simulink model "BLDCmotorControl_FOC_R2017b"  (R2017b)
settings: Solver=FixedStepDiscrete  StartTime=0  StopTime=1  FixedStep=Ts  MaxStep=1e-6  RelTol=1e-6  AbsTol=1e-6  EnableMultiTasking=on
PreLoadFcn:
  | addpath(genpath('01_Libraries'));
  | addpath(genpath('02_Figures'));
InitFcn:
  | init_model;
values from neighbouring files (symbols this model uses):
  a_elecAngle = 60    [init_model_Ffwd.m]
  a_elecPeriod = 360    [init_model_Ffwd.m]
  b_DCLinkCurrAvail = 0    [init_model_Ffwd.m]
  b_selPhaABCurrMeas = 1    [init_model_Ffwd.m]
  cf_speedCoef = round(f_ctrl * a_mechAngle * (pi/180) * (30/pi))    [init_model_Ffwd.m]
  i_thresOutlier = 200    [init_model_Ffwd.m]
  n_commAcvLo = 15    [init_model_Ffwd.m]
  n_commDeacvHi = 30    [init_model_Ffwd.m]
  r_sin_M1 = sin((a_elecAngle_XA + 30)*(pi/180))    [init_model_Ffwd.m]
  r_whl = 6.5 * 2.54 * 1e-2 / 2    (= 0.08255)    [init_model_Ffwd.m]
  res_elecAngle = 2    [init_model_Ffwd.m]
  Ts = 5e-6    (= 5e-06)    [init_model_Ffwd.m]    (also in pe_electric_engine_dyno_data.m = 1e-05)
  Ts_ctrl = 6e-5    (= 6e-05)    [init_model_Ffwd.m]
  vec_hallToPos = [0 2 0 1 4 3 5 0]    [init_model_Ffwd.m]
  z_commutMap_M1 = [-1 -1  0  1  1  0 ... (first row only)    [init_model_Ffwd.m]
  z_ctrlTypSel = 1    [init_model_Ffwd.m]
  z_maxCntRst = 2000    [init_model_Ffwd.m]
undefined symbols (not defined in the file or in its folder): a_phaAdv_M1, b_phaAdvEna, CTRL_COMM, DiscIntNeverNeededParam, Down, dz_counterHi, dz_counterLo, Kb_Id, Kb_Iq, Kb_n, Ki_Id, Ki_Iq, Ki_n, Kp_Id, Kp_Iq, Kp_n, n_motPhaAdvEna, r_commDCDeacv, sigbuilder_block, Up, V_circleLim_M1, V_max, V_min
libraries: pePwmGenerator x7, BLDC_controller_Lib x6, powerlib x6, simulink x5
(part 3 of 3)

== system BLDCmotorControl_FOC_R2017b/BLDC_controller/BLDC_controller/F03_Field_Oriented_Control/Clarke_Transform/Clarke_PhasesAB ==
  note: Clarke Transform:
      | i_alpha = i_phaA
      | i_beta = ((1/sqrt(3))*i_phaA + (2/sqrt(3))*i_phaB)
  i_phaA : Inport
  i_phaB : Inport  Port=2
  Action Port : ActionPort  ActionType=then
  Gain1 : Gain  Tag=struct('comment',struct('text','','placement',1),'logdata',struct('maxnumvals',inf,'plotchannels',[],'loggingmode',3,'channels',1),'output',struct('variable','','description','','name','$S_$B','width',1,'address','','max',NaN,'min',NaN,'class','default','type','CONTINUOUS','scaling','','lsb',1,'offset',0,'arb',0,'freeze',1,'unit','','autoscalingmode',1,'lowerheadroom',1,'upperheadroom',1,'headroomunit','bit','keepdatatype',1,'checkmin',0,'checkmax',0,'castoutput',0,'show',0),'gain',struct('variable','','description','','name','$S_$B_gain','width',1,'address','','max',NaN,'min',NaN,'class','default','type','CONTINUOUS','scaling','','lsb',1,'offset',0,'arb',0,'freeze',1,'unit','','keepdatatype',1,'value','1','scalar',0,'tolerance',1),'scalingvalid',0,'date',730486)  Gain=2/sqrt(3)  RndMeth=Zero
  Gain3 : Gain  Tag=struct('comment',struct('text','','placement',1),'logdata',struct('maxnumvals',inf,'plotchannels',[],'loggingmode',3,'channels',1),'output',struct('variable','','description','','name','$S_$B','width',1,'address','','max',NaN,'min',NaN,'class','default','type','CONTINUOUS','scaling','','lsb',1,'offset',0,'arb',0,'freeze',1,'unit','','autoscalingmode',1,'lowerheadroom',1,'upperheadroom',1,'headroomunit','bit','keepdatatype',1,'checkmin',0,'checkmax',0,'castoutput',0,'show',0),'gain',struct('variable','','description','','name','$S_$B_gain','width',1,'address','','max',NaN,'min',NaN,'class','default','type','CONTINUOUS','scaling','','lsb',1,'offset',0,'arb',0,'freeze',1,'unit','','keepdatatype',1,'value','1','scalar',0,'tolerance',1),'scalingvalid',0,'date',730486)  Gain=1/sqrt(3)  RndMeth=Zero
  Sum6 : Sum  RndMeth=Simplest
  for_merge : Gain  Tag=struct('comment',struct('text','','placement',1),'logdata',struct('maxnumvals',inf,'plotchannels',[],'loggingmode',3,'channels',1),'output',struct('variable','','description','','name','$S_$B','width',1,'address','','max',NaN,'min',NaN,'class','default','type','CONTINUOUS','scaling','','lsb',1,'offset',0,'arb',0,'freeze',1,'unit','','autoscalingmode',1,'lowerheadroom',1,'upperheadroom',1,'headroomunit','bit','keepdatatype',1,'checkmin',0,'checkmax',0,'castoutput',0,'show',0),'gain',struct('variable','','description','','name','$S_$B_gain','width',1,'address','','max',NaN,'min',NaN,'class','default','type','CONTINUOUS','scaling','','lsb',1,'offset',0,'arb',0,'freeze',1,'unit','','keepdatatype',1,'value','1','scalar',0,'tolerance',1),'scalingvalid',0,'date',730486)  RndMeth=Zero
  i_alphaAB : Outport
  i_betaAB : Outport  Port=2
  wires:
  i_phaB/1 -> [i_phaB]
  i_phaA/1 -> [i_phaA]
  [i_phaB] -> Gain1/1
  [i_phaA] -> for_merge/1, Gain3/1
  Gain3/1 -> Sum6/1
  Sum6/1 -> i_betaAB/1  "beta"
  Gain1/1 -> Sum6/2
  for_merge/1 -> i_alphaAB/1

== system BLDCmotorControl_FOC_R2017b/BLDC_controller/BLDC_controller/F03_Field_Oriented_Control/Clarke_Transform/Clarke_PhasesBC ==
  note: Clarke Transform:
      | i_alpha = - i_phaB - i_phaC
      | i_beta = (1/sqrt(3)) * (i_phaB - i_phaC)
  i_phaB : Inport
  i_phaC : Inport  Port=2
  Action Port : ActionPort  ActionType=else
  Gain2 : Gain  Tag=struct('comment',struct('text','','placement',1),'logdata',struct('maxnumvals',inf,'plotchannels',[],'loggingmode',3,'channels',1),'output',struct('variable','','description','','name','$S_$B','width',1,'address','','max',NaN,'min',NaN,'class','default','type','CONTINUOUS','scaling','','lsb',1,'offset',0,'arb',0,'freeze',1,'unit','','autoscalingmode',1,'lowerheadroom',1,'upperheadroom',1,'headroomunit','bit','keepdatatype',1,'checkmin',0,'checkmax',0,'castoutput',0,'show',0),'gain',struct('variable','','description','','name','$S_$B_gain','width',1,'address','','max',NaN,'min',NaN,'class','default','type','CONTINUOUS','scaling','','lsb',1,'offset',0,'arb',0,'freeze',1,'unit','','keepdatatype',1,'value','1','scalar',0,'tolerance',1),'scalingvalid',0,'date',730486)  Gain=1/sqrt(3)  RndMeth=Zero
  Sum1 : Sum  Inputs=--  RndMeth=Simplest
  Sum2 : Sum  Inputs=+-  RndMeth=Simplest
  i_alphaBC : Outport
  i_betaBC : Outport  Port=2
  wires:
  [i_phaC] -> Sum1/2
  [i_phaB] -> Sum1/1
  [i_phaC] -> Sum2/2
  Gain2/1 -> i_betaBC/1
  Sum2/1 -> Gain2/1
  [i_phaB] -> Sum2/1
  Sum1/1 -> i_alphaBC/1
  i_phaB/1 -> [i_phaB]
  i_phaC/1 -> [i_phaC]

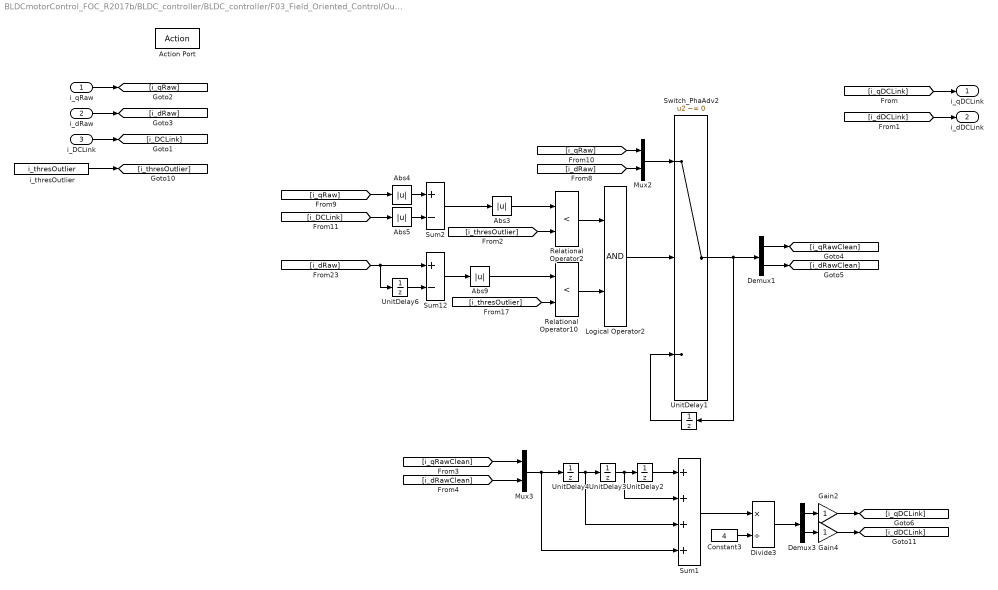
== system BLDCmotorControl_FOC_R2017b/BLDC_controller/BLDC_controller/F03_Field_Oriented_Control/Outliers_Removal/DCLink_Current_Available ==
  i_qRaw : Inport
  i_dRaw : Inport  Port=2
  i_DCLink : Inport  Port=3
  Action Port : ActionPort  ActionType=then
  Abs{3..5,9} (4 alike) : Abs
  Constant3 : Constant  Value=4  OutDataTypeStr=Inherit: Inherit via back propagation
  Demux1 : Demux  Outputs=2
  Demux3 : Demux  Outputs=2
  Divide3 : Product  Inputs=*/  RndMeth=Simplest
  Gain2 : Gain  Tag=struct('comment',struct('text','','placement',1),'logdata',struct('maxnumvals',inf,'plotchannels',[],'loggingmode',3,'channels',1),'output',struct('variable','','description','','name','$S_$B','width',1,'address','','max',NaN,'min',NaN,'class','default','type','CONTINUOUS','scaling','','lsb',1,'offset',0,'arb',0,'freeze',1,'unit','','autoscalingmode',1,'lowerheadroom',1,'upperheadroom',1,'headroomunit','bit','keepdatatype',1,'checkmin',0,'checkmax',0,'castoutput',0,'show',0),'gain',struct('variable','','description','','name','$S_$B_gain','width',1,'address','','max',NaN,'min',NaN,'class','default','type','CONTINUOUS','scaling','','lsb',1,'offset',0,'arb',0,'freeze',1,'unit','','keepdatatype',1,'value','1','scalar',0,'tolerance',1),'scalingvalid',0,'date',730486)  RndMeth=Zero  SaturateOnIntegerOverflow=on  OutDataTypeStr=Inherit: Same as input  ParamDataTypeStr=Inherit: Same as input
  Gain4 : Gain  Tag=struct('comment',struct('text','','placement',1),'logdata',struct('maxnumvals',inf,'plotchannels',[],'loggingmode',3,'channels',1),'output',struct('variable','','description','','name','$S_$B','width',1,'address','','max',NaN,'min',NaN,'class','default','type','CONTINUOUS','scaling','','lsb',1,'offset',0,'arb',0,'freeze',1,'unit','','autoscalingmode',1,'lowerheadroom',1,'upperheadroom',1,'headroomunit','bit','keepdatatype',1,'checkmin',0,'checkmax',0,'castoutput',0,'show',0),'gain',struct('variable','','description','','name','$S_$B_gain','width',1,'address','','max',NaN,'min',NaN,'class','default','type','CONTINUOUS','scaling','','lsb',1,'offset',0,'arb',0,'freeze',1,'unit','','keepdatatype',1,'value','1','scalar',0,'tolerance',1),'scalingvalid',0,'date',730486)  RndMeth=Zero  SaturateOnIntegerOverflow=on  OutDataTypeStr=Inherit: Same as input  ParamDataTypeStr=Inherit: Same as input
  Logical Operator2 : Logic  AllPortsSameDT=off  OutDataTypeStr=boolean
  Mux2 : Mux  Inputs=2
  Mux3 : Mux  Inputs=2
  Relational Operator10 : RelationalOperator  Operator=<  OutDataTypeStr=boolean  RndMeth=Simplest
  Relational Operator2 : RelationalOperator  Operator=<  OutDataTypeStr=boolean  RndMeth=Simplest
  Sum1 : Sum  Inputs=++++  RndMeth=Simplest  InputSameDT=on
  Sum12 : Sum  Inputs=+-  RndMeth=Simplest
  Sum2 : Sum  Inputs=+-  RndMeth=Simplest
  Switch_PhaAdv2 : Switch  Criteria=u2 ~= 0  OutDataTypeStr=Inherit: Inherit via back propagation  RndMeth=Zero
  UnitDelay{1..4,6} (5 alike) : UnitDelay  SampleTime=-1
  i_thresOutlier : Constant  Value=i_thresOutlier  OutDataTypeStr=Inherit: Inherit via back propagation
  i_qDCLink : Outport
  i_dDCLink : Outport  Port=2
  wires:
  [i_dDCLink] -> i_dDCLink/1
  i_qRaw/1 -> [i_qRaw]
  [i_qDCLink] -> i_qDCLink/1
  i_dRaw/1 -> [i_dRaw]
  i_DCLink/1 -> [i_DCLink]
  Switch_PhaAdv2/1 -> Demux1/1, UnitDelay1/1
  Mux2/1 -> Switch_PhaAdv2/1
  Logical Operator2/1 -> Switch_PhaAdv2/2
  [i_DCLink] -> Abs5/1
  UnitDelay6/1 -> Sum12/2
  Demux1/1 -> [i_qRawClean]
  [i_thresOutlier] -> Relational Operator2/2
  Relational Operator10/1 -> Logical Operator2/2
  [i_dRaw] -> Mux2/2
  Abs9/1 -> Relational Operator10/1
  [i_thresOutlier] -> Relational Operator10/2
  Abs5/1 -> Sum2/2
  [i_dRaw] -> UnitDelay6/1, Sum12/1
  Abs3/1 -> Relational Operator2/1
  Demux1/2 -> [i_dRawClean]
  UnitDelay1/1 -> Switch_PhaAdv2/3
  [i_qRaw] -> Abs4/1
  [i_qRaw] -> Mux2/1
  Abs4/1 -> Sum2/1
  Relational Operator2/1 -> Logical Operator2/1
  Sum2/1 -> Abs3/1
  Sum12/1 -> Abs9/1
  Demux3/2 -> Gain4/1
  Gain2/1 -> [i_qDCLink]
  Divide3/1 -> Demux3/1
  Mux3/1 -> Sum1/4, UnitDelay4/1
  Gain4/1 -> [i_dDCLink]
  UnitDelay4/1 -> Sum1/3, UnitDelay3/1
  [i_qRawClean] -> Mux3/1
  Sum1/1 -> Divide3/1
  UnitDelay3/1 -> Sum1/2, UnitDelay2/1
  Constant3/1 -> Divide3/2
  UnitDelay2/1 -> Sum1/1
  Demux3/1 -> Gain2/1
  [i_dRawClean] -> Mux3/2
  i_thresOutlier/1 -> [i_thresOutlier]

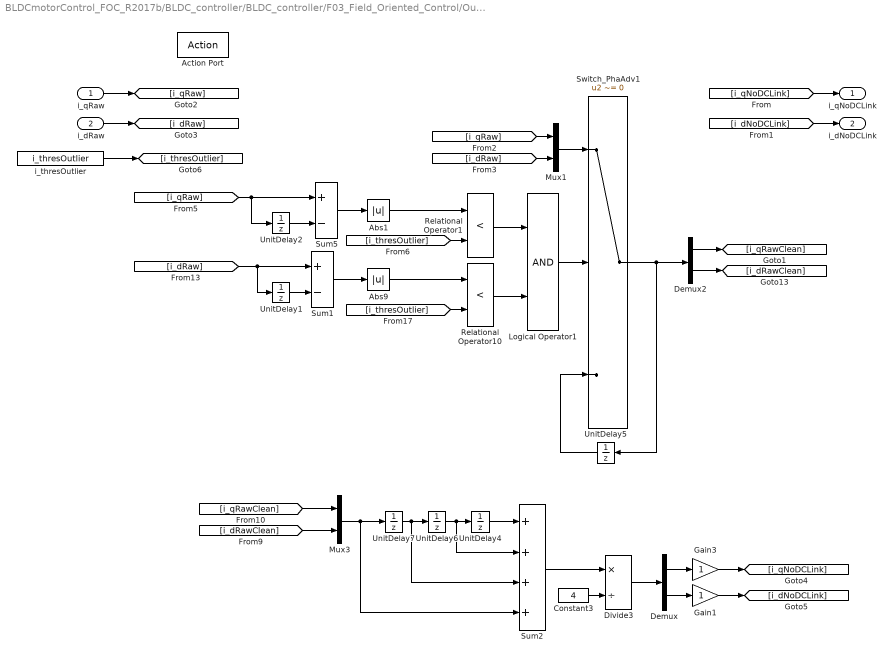
== system BLDCmotorControl_FOC_R2017b/BLDC_controller/BLDC_controller/F03_Field_Oriented_Control/Outliers_Removal/DCLink_Current_Not_Available ==
  i_qRaw : Inport
  i_dRaw : Inport  Port=2
  Action Port : ActionPort  ActionType=else
  Abs1 : Abs
  Abs9 : Abs
  Constant3 : Constant  Value=4  OutDataTypeStr=Inherit: Inherit via back propagation
  Demux : Demux  Outputs=2
  Demux2 : Demux  Outputs=2
  Divide3 : Product  Inputs=*/  RndMeth=Simplest
  Gain1 : Gain  Tag=struct('comment',struct('text','','placement',1),'logdata',struct('maxnumvals',inf,'plotchannels',[],'loggingmode',3,'channels',1),'output',struct('variable','','description','','name','$S_$B','width',1,'address','','max',NaN,'min',NaN,'class','default','type','CONTINUOUS','scaling','','lsb',1,'offset',0,'arb',0,'freeze',1,'unit','','autoscalingmode',1,'lowerheadroom',1,'upperheadroom',1,'headroomunit','bit','keepdatatype',1,'checkmin',0,'checkmax',0,'castoutput',0,'show',0),'gain',struct('variable','','description','','name','$S_$B_gain','width',1,'address','','max',NaN,'min',NaN,'class','default','type','CONTINUOUS','scaling','','lsb',1,'offset',0,'arb',0,'freeze',1,'unit','','keepdatatype',1,'value','1','scalar',0,'tolerance',1),'scalingvalid',0,'date',730486)  RndMeth=Zero  SaturateOnIntegerOverflow=on  OutDataTypeStr=Inherit: Same as input  ParamDataTypeStr=Inherit: Same as input
  Gain3 : Gain  Tag=struct('comment',struct('text','','placement',1),'logdata',struct('maxnumvals',inf,'plotchannels',[],'loggingmode',3,'channels',1),'output',struct('variable','','description','','name','$S_$B','width',1,'address','','max',NaN,'min',NaN,'class','default','type','CONTINUOUS','scaling','','lsb',1,'offset',0,'arb',0,'freeze',1,'unit','','autoscalingmode',1,'lowerheadroom',1,'upperheadroom',1,'headroomunit','bit','keepdatatype',1,'checkmin',0,'checkmax',0,'castoutput',0,'show',0),'gain',struct('variable','','description','','name','$S_$B_gain','width',1,'address','','max',NaN,'min',NaN,'class','default','type','CONTINUOUS','scaling','','lsb',1,'offset',0,'arb',0,'freeze',1,'unit','','keepdatatype',1,'value','1','scalar',0,'tolerance',1),'scalingvalid',0,'date',730486)  RndMeth=Zero  SaturateOnIntegerOverflow=on  OutDataTypeStr=Inherit: Same as input  ParamDataTypeStr=Inherit: Same as input
  Logical Operator1 : Logic  AllPortsSameDT=off  OutDataTypeStr=boolean
  Mux1 : Mux  Inputs=2
  Mux3 : Mux  Inputs=2
  Relational Operator1 : RelationalOperator  Operator=<  OutDataTypeStr=boolean  RndMeth=Simplest
  Relational Operator10 : RelationalOperator  Operator=<  OutDataTypeStr=boolean  RndMeth=Simplest
  Sum1 : Sum  Inputs=+-  RndMeth=Simplest
  Sum2 : Sum  Inputs=++++  RndMeth=Simplest  InputSameDT=on
  Sum5 : Sum  Inputs=+-  RndMeth=Simplest
  Switch_PhaAdv1 : Switch  Criteria=u2 ~= 0  OutDataTypeStr=Inherit: Inherit via back propagation  RndMeth=Zero
  UnitDelay{1..2,4..7} (6 alike) : UnitDelay  SampleTime=-1
  i_thresOutlier : Constant  Value=i_thresOutlier  OutDataTypeStr=Inherit: Inherit via back propagation
  i_qNoDCLink : Outport
  i_dNoDCLink : Outport  Port=2
  wires:
  i_qRaw/1 -> [i_qRaw]
  i_dRaw/1 -> [i_dRaw]
  [i_qNoDCLink] -> i_qNoDCLink/1
  [i_dNoDCLink] -> i_dNoDCLink/1
  Logical Operator1/1 -> Switch_PhaAdv1/2
  Constant3/1 -> Divide3/2
  UnitDelay6/1 -> Sum2/2, UnitDelay4/1
  UnitDelay7/1 -> Sum2/3, UnitDelay6/1
  [i_qRawClean] -> Mux3/1
  Sum1/1 -> Abs9/1
  Abs9/1 -> Relational Operator10/1
  [i_dRaw] -> UnitDelay1/1, Sum1/1
  Sum2/1 -> Divide3/1
  [i_thresOutlier] -> Relational Operator10/2
  Divide3/1 -> Demux/1
  Demux2/1 -> [i_qRawClean]
  Demux/1 -> Gain3/1
  Demux2/2 -> [i_dRawClean]
  Relational Operator10/1 -> Logical Operator1/2
  UnitDelay1/1 -> Sum1/2
  Abs1/1 -> Relational Operator1/1
  Gain3/1 -> [i_qNoDCLink]
  [i_qRaw] -> Mux1/1
  Sum5/1 -> Abs1/1
  [i_thresOutlier] -> Relational Operator1/2
  Gain1/1 -> [i_dNoDCLink]
  Mux3/1 -> Sum2/4, UnitDelay7/1
  Mux1/1 -> Switch_PhaAdv1/1
  Switch_PhaAdv1/1 -> Demux2/1, UnitDelay5/1
  UnitDelay4/1 -> Sum2/1
  [i_dRaw] -> Mux1/2
  UnitDelay2/1 -> Sum5/2
  UnitDelay5/1 -> Switch_PhaAdv1/3
  Relational Operator1/1 -> Logical Operator1/1
  [i_qRaw] -> Sum5/1, UnitDelay2/1
  [i_dRawClean] -> Mux3/2
  Demux/2 -> Gain1/1
  i_thresOutlier/1 -> [i_thresOutlier]
